simulink model "experimentident"  (R2019b)
settings: Solver=VariableStepAuto  StartTime=0.0  StopTime=30  RelTol=1e-3
values from neighbouring files (symbols this model uses):
  den = [1,5,8]    [FinalAlgorithm.m]
  num = 1    [FinalAlgorithm.m]
  ts = 1e-1    (= 0.1)    [FinalAlgorithm.m]
settings Model: Creator=adrian  LastModifiedBy=adrian

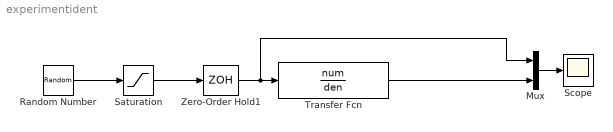
== system experimentident ==
  Mux : Mux  Inputs=2
  Random Number : RandomNumber  SampleTime=1
  Saturation : Saturate  UpperLimit=5  LowerLimit=0
  Scope : Scope
  Transfer Fcn : TransferFcn  Numerator=num  Denominator=den
  Zero-Order Hold1 : ZeroOrderHold  SampleTime=ts
  wires:
  Mux/1 -> Scope/1
  Transfer Fcn/1 -> Mux/2
  Zero-Order Hold1/1 -> Mux/1, Transfer Fcn/1
  Random Number/1 -> Saturation/1
  Saturation/1 -> Zero-Order Hold1/1
